simulink model "Amplitude_modulation_simulink"  (R2020b)
settings: Solver=VariableStepAuto  StartTime=0.0  StopTime=10.0  RelTol=1e-3
libraries: dspfdesign x1
settings Model: Creator=Arnab Das  LastModifiedBy=Arnab Das

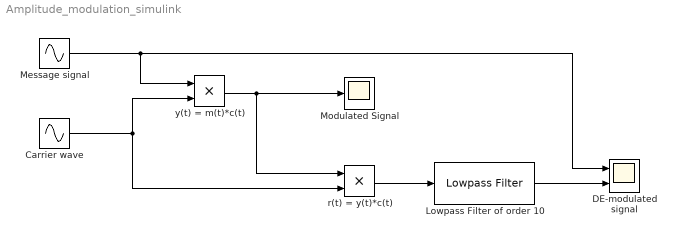
== system Amplitude_modulation_simulink ==
  Carrier wave : Sin  Frequency=10000  SampleTime=0.01
  DE-modulated signal : Scope  NumInputPorts=2
  Lowpass Filter of order 10 : dspfdesign/Lowpass Filter  FilterType=FIR  DesignForMinimumOrder=on  FilterOrder=50  PassbandFrequency=10  StopbandFrequency=15  PassbandRipple=0.01  StopbandAttenuation=180  InheritSampleRate=off  SampleRate=100  SimulateUsing=Interpreted execution  roundingMode=Floor  coeffsDataTypeStr=fixdt(1,16)
  Message signal : Sin  Frequency=10  SampleTime=0.01
  Modulated Signal : Scope
  r(t) = y(t)*c(t) : Product
  y(t) = m(t)*c(t) : Product
  wires:
  y(t) = m(t)*c(t)/1 -> Modulated Signal/1, r(t) = y(t)*c(t)/1
  Message signal/1 -> DE-modulated signal/1, y(t) = m(t)*c(t)/1
  Carrier wave/1 -> r(t) = y(t)*c(t)/2, y(t) = m(t)*c(t)/2
  r(t) = y(t)*c(t)/1 -> Lowpass Filter of order 10/1
  Lowpass Filter of order 10/1 -> DE-modulated signal/2
